simulink model "forward_invers_kinematics_validation"  (R2019b)
settings: Solver=VariableStepAuto  StartTime=0.0  StopTime=10.0  RelTol=1e-3
settings Model: Creator=Trygg  LastModifiedBy=Trygg

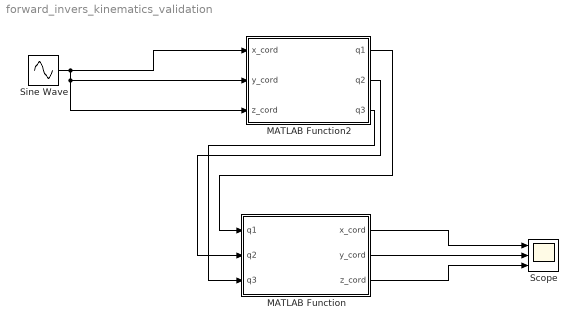
== system forward_invers_kinematics_validation ==
  MATLAB Function : MATLAB Function  Tag=Forward Kinematics  Description=Forward kinematics block  TreatAsAtomicUnit=on
  MATLAB Function2 : MATLAB Function  TreatAsAtomicUnit=on
  Scope : Scope  NumInputPorts=3
  Sine Wave : Sin  Amplitude=500  SampleTime=0
  wires:
  MATLAB Function2/1(q1) -> MATLAB Function/1(q1)
  MATLAB Function2/2(q2) -> MATLAB Function/2(q2)
  MATLAB Function2/3(q3) -> MATLAB Function/3(q3)
  MATLAB Function/1(x_cord) -> Scope/1
  MATLAB Function/2(y_cord) -> Scope/2
  MATLAB Function/3(z_cord) -> Scope/3
  Sine Wave/1 -> MATLAB Function2/3(z_cord), MATLAB Function2/2(y_cord), MATLAB Function2/1(x_cord)

== matlab function forward_invers_kinematics_validation/MATLAB Function ==
  data: q1 input; q2 input; x_cord output; q3 input; y_cord output; z_cord output
% 
% %Foreward kinematics function
 function [x_cord, y_cord, z_cord]= ForwardKinematics(q1, q2, q3)
% 
% %_______________Data Given______________________
% L1= 0;   %0.128;  %0.85; %Length o f the f i r s t l i n k
% L2= 1;   %06177;  %0.5; %Length o f the second l i n k
% L3= 1;   %0.5716;  %0.35; %Length og the thi rd l i n k
% 
% c1=cos(q1);
% c2=cos(q2);
% c23=cos(q2+q3);
% 
% s1=sin(q1);
% s2=sin(q2);
% s23=sin(q2+q3);
% 
% %_______________End−e f f e c t o r position______________________
% 
% % x=c0*(L2*c1+L3*c12) ;
% % y=s0*(L2*c1+L3*c12);
% % z=L1+L2*s1+L3*s12;
% x = c1*c23*L3+c1*c2*L2;
% y = s1*c23*L3+s1*c2*L2;
% z = s23*L3+s2*L2+L1;

%format short g

%%%%%PARAMETERS%%%%%%%%%DH matrix
alpha =  [0 pi/2 0 0];
d = [0.1273 0 0 0]*1000; %.0127
a = [0 0 -0.612 -0.688]*1000;
%Decired angles 
theta = [q1 0  q2 q3];



T0 = [cos(theta(1)) -sin(theta(1))*cos(alpha(1)) sin(theta(1))*sin(alpha(1)) a(1)*cos(theta(1));
          sin(theta(1)) cos(theta(1))*cos(alpha(1)) -cos(theta(1))*sin(alpha(1)) a(1)*sin(theta(1));
          0 sin(alpha(1)) cos(alpha(1)) d(1);
          0 0 0 1];

T1 = [cos(theta(2)) -sin(theta(2))*cos(alpha(2)) sin(theta(2))*sin(alpha(2)) a(2)*cos(theta(2));
      sin(theta(2)) cos(theta(2))*cos(alpha(2)) -cos(theta(2))*sin(alpha(2)) a(2)*sin(theta(2));
      0 sin(alpha(2)) cos(alpha(2)) d(2);
      0 0 0 1];

T2 = [cos(theta(3)) -sin(theta(3))*cos(alpha(3)) sin(theta(3))*sin(alpha(3)) a(3)*cos(theta(3));
      sin(theta(3)) cos(theta(3))*cos(alpha(3)) -cos(theta(3))*sin(alpha(3)) a(3)*sin(theta(3));
      0 sin(alpha(3)) cos(alpha(3)) d(3);
      0 0 0 1];
T3 = [cos(theta(4)) -sin(theta(4))*cos(alpha(4)) sin(theta(4))*sin(alpha(4)) a(4)*cos(theta(4));
      sin(theta(4)) cos(theta(4))*cos(alpha(4)) -cos(theta(4))*sin(alpha(4)) a(4)*sin(theta(4));
      0 sin(alpha(4)) cos(alpha(4)) d(4);
      0 0 0 1];

T4= T0*T1*T2*T3;
%phi = theta(3) + theta(4) - pi



x_cord = T4(1,4)
y_cord = T4(2,4)
z_cord = T4(3,4)

== matlab function forward_invers_kinematics_validation/MATLAB Function2 ==
  data: q1 output; q2 output; q3 output; x_cord input; y_cord input; z_cord input
% % 
% % %Inverse kinematics function
% % 
function[q1, q2, q3]= InverseKinematics(x_cord, y_cord, z_cord)
% % 
% % 
% % %_______________Data Given______________________
% % 
% % L1= 0; %0.128;  %0.85; %Length o f the f i r s t l i n k
% % L2= 1; %06177;  %0.5; %Length o f the second l i n k
% % L3= 1; %0.5716;  %0.35; %Length og the thi rd l i n k
% % %r = x.^2+y.^2+z.^2;
% % %q0 = base
% % %q1 = shoulder
% % %q2 = elbow
% % 
% % %c2=cos(q2);
% % %c23=cos(q2+q3);
% % 
% % 
% % %s2=sin(q2);
% % %s23=sin(q2+q3);
% % 
% % 
% % 
% % %q1 = atan2(y,x);
% % %c1=cos(q1);
% % %s1=sin(q1);
% % %c3 = (x^2+y^2+z^2-(L1^2+L2^2+L3^2)-2*L1*(z-L1))/(2*L2*L3);
% % %s3p = sqrt(1-c3);
% % %s3n = -sqrt(1-c3);
% % %Check if equation contain imaginary value
% % %if real(s3p) == 0
% %     %s3p = 0;
% % %end
% % %if real(s3n) == 0
% %     %s3n = 0;
% % %end
% % %s3p = real(s3p);
% % %s3n = real(s3n);
% % %a = (z-L1)*(c1-s1);
% % %b = (x-y);
% % %c = s3p*L3;
% % %d = c3*L3+L2;
% % %q21 = atan2(a,b)-atan2(c,d);
% % %q31 = atan2(s3p,c3);
% % %q22 = atan2((z-L1)*(c1-s1),(x-y))-atan2(s3n*L3,c3*L3+L2);
% % %q32 = atan2(s3n,c3);
% % 
% % q1 = atan2(y,x);
% % while q1 <0
% %     
% %     q1 = q1 +pi;
% % end
% % 
% % while q1 > pi
% %     q1 = q1-pi;
% % end
% % 
% % %display(q1);
% % 
% % c1=cos(q1);
% % s1=sin(q1);
% % c3 = (x^2+y^2+z^2-(L1^2+L2^2+L3^2)-2*L1*(z-L1))/(2*L2*L3);
% % s3p = sqrt(1-c3);
% % s3n = -sqrt(1-c3);
% % %Check if equation contain imaginary value
% % %if real(s3p) == 0
% %     %s3p = 0;
% % %end
% % %if real(s3n) == 0
% %     %s3n = 0;
% % %end
% % %s3p = real(s3p);
% % %s3n = real(s3n);
% % a = (z-L1)*(c1-s1);
% % b = (x-y);
% % c = s3p*L3;
% % d = c3*L3+L2;
% % e = s3n*L3;
% % q21 = atan2(a,b)-atan2(c,d);
% % q31 = atan2(s3p,c3);
% % q22 = atan2(a,b)-atan2(e,d);
% % q32 = atan2(s3n,c3);
% % %q22 = atan2((z-L1)*(c1-s1),(x-y))-atan2(s3n*L3,c3*L3+L2)
% % q2 = q22;
% % q3= q32;
% % 
% % if q31 < 0
% %     q3 = q31;
% %     q2 = q21;
% % end
% % if q32 <0
% %     q3 = q32;
% %     q2 = q22;
% % end
% % 
% % 
% % 
% % if abs(q1)<1e-6
% %    q1=0;
% % end
% % if abs(q21)<1e-6
% %    q21=0;
% % end
% % if abs(q31)<1e-6
% %    q31=0;
% % end
% % if abs(q22)<1e-6
% %    q22=0;
% % end
% % if abs(q32)<1e-6
% %    q32=0;
% % end
% % if abs(q3)<1e-6
% %    q3=0;
% % end
% % if abs(q2)<1e-6
% %    q2=0;
% % end
% % 
% % 
% % 
% % 
% %syms theta_0 theta_1 theta_2
% %format short g
% 
% offset = [0 0 0 0];
% alpha =  [0 pi/2 0 0];
% % d = [0.128 0 0 0.0125]*1000;
% % a = [0 0 -0.612 -0.68759]*1000;
% d = [0.128 0 0 0]*1000;
% a = [0 0 0.612 0.6875]*1000;
% 
% 
% 
% s3pn = 1;
% q2pn = -1;
% q1 = atan2(y_cord,x_cord);
% % if y_cord >= 0
% %     q1 = q1 - pi;
% % else
% %     q1 = q1 + pi;
% % end
% 
% c3 = ((x_cord^2+y_cord^2+z_cord^2-(d(1)^2+a(3)^2+a(4)^2)-2*d(1)*(z_cord-d(1)))/(2*a(3)*a(4)))
% s3 = real(s3pn*sqrt(1-c3))
% 
% 
% q3 = atan2(s3,c3)
% %q2b = atan2(((z_cord-d(1))*(cos(q1)-sin(q1))),(x_cord-y_cord))-atan2(s3*a(4),(c3*a(4)+a(3))); %LÃ¸sning 1
% 
%  %__________________________LÃ¸sning 2_____________________________%
% k1 = c3*a(4)+a(3)
% k2 = s3*a(4)
% 
% A = -2*k1*(d(1)-z_cord)
% B = (2*k1*(d(1)-z_cord))^2-4*(k1^2+k2^2)*(z_cord^2+d(1)^2-k2^2-2*z_cord*d(1))
% q2 = asin((A+q2pn*sqrt(B))/(2*(k1^2+k2^2)))
% q2 = real(q2)
% R=sqrt(x_cord^2+y_cord^2);

alpha =  [0 pi/2 0 0];  %Joint Angle offset
d = [0.1273 0 0 0]*1000;  %0.0127   Link offset
a = [0 0 0.612 0.688]*1000;   %LINK LENGTH   %-0.5723-0.1157 =-0.688

%Defined geometric properties
R=sqrt(x_cord^2+y_cord^2);
L = sqrt(d(1)^2+R^2);

%%%%%%%%%First equations%%%%%%%
q1 = atan2(y_cord,x_cord); %Base

%limit possibilities for base%
if y_cord <= 0
    q1 = q1 + pi;
else
    q1 = q1 - pi;
end

 

%calculate r1,r2,r3
r1 = sqrt(x_cord^2+y_cord^2);
r2 = z_cord-d(1);
r3 = sqrt(r2^2+r1^2);

%calculate pi1,pi2,pi3
pi1 = -atan2(r2,r1);
 
pi2 = -acos(((a(3)^2)+(r3^2)-(a(4)^2))/(2*a(3)*r3));
 
pi3 = acos(((a(3)^2)+(a(4)^2)-(r3^2))/(2*a(3)*a(4)));
 
%calculate theta1,theta2,theta3

q2 = real(pi1+pi2);
q3 = real(pi-pi3);
